simulink library "purePursuitCtrl_cl"  (R2018b)
settings: Solver=VariableStepAuto  StartTime=0.0  StopTime=10.0  RelTol=1e-3
values from neighbouring files (symbols this model uses):
  numberOfLaps_none = 5    [purePursuitCtrl_cl_init.m]
libraries: simulink x1, headingSetpointCalculation_cl x1, lapCounter_ul x1
settings Model: Creator=mcobb  LastModifiedBy=mcobb
settings DebuggingCC: LibraryContextMissingDiagnostic=none
settings SFSimCC: SimUseLocalCustomCode=off
settings RTWCC: RTWUseLocalCustomCode=off

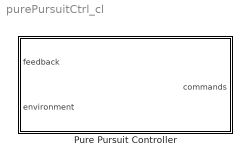
== system purePursuitCtrl_cl ==
  Pure Pursuit Controller : Subsystem  VariantControl=VSS_PUREPURSUIT_CTRL

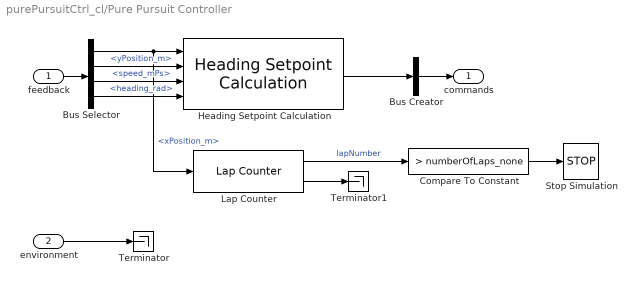
== system purePursuitCtrl_cl/Pure Pursuit Controller ==
  feedback : Inport
  environment : Inport  Port=2
  Bus Creator : BusCreator  Inputs=1
  Bus Selector : BusSelector  OutputSignals=xPosition_m,yPosition_m,speed_mPs,heading_rad
  Compare To Constant : simulink/Logic and Bit Operations/Compare To Constant  relop=>  const=numberOfLaps_none  OutDataTypeStr=boolean
  Heading Setpoint Calculation : headingSetpointCalculation_cl/Heading Setpoint Calculation  SystemSampleTime=-1
  Lap Counter : lapCounter_ul/Lap Counter  SystemSampleTime=-1
  Stop Simulation : Stop
  Terminator : Terminator
  Terminator1 : Terminator
  commands : Outport
  wires:
  Bus Selector/4 -> Heading Setpoint Calculation/4  "<heading_rad>"
  Bus Selector/3 -> Heading Setpoint Calculation/3  "<speed_mPs>"
  feedback/1 -> Bus Selector/1
  Bus Selector/1 -> Heading Setpoint Calculation/1, Lap Counter/1  "<xPosition_m>"
  Bus Selector/2 -> Heading Setpoint Calculation/2  "<yPosition_m>"
  environment/1 -> Terminator/1
  Heading Setpoint Calculation/1 -> Bus Creator/1
  Bus Creator/1 -> commands/1
  Lap Counter/1 -> Compare To Constant/1  "lapNumber"
  Compare To Constant/1 -> Stop Simulation/1
  Lap Counter/2 -> Terminator1/1
